simulink model "simulacao"  (R2025a)
settings: Solver=VariableStepAuto  StartTime=0.0  StopTime=50  RelTol=1e-3
undefined symbols (not defined in the file): b, g, J, l, m, Tc, theta0_rad
settings Model: Creator=luiza  LastModifiedBy=luiza

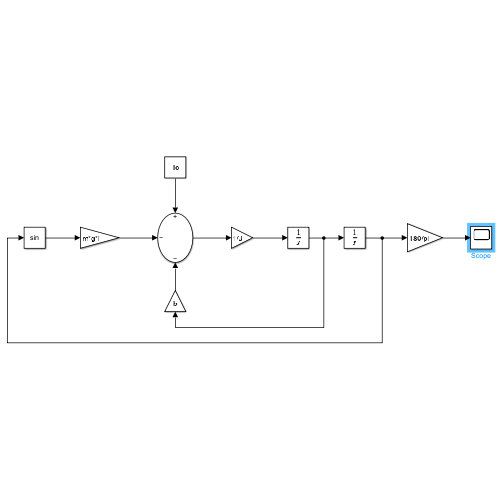
[thumbnail: Simulink's stored preview of the top-level diagram]
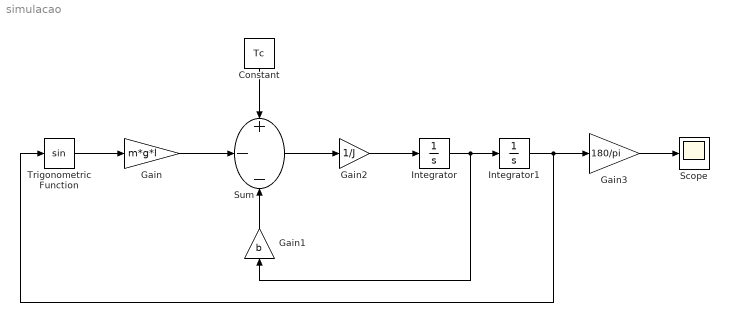
== system simulacao ==
  Constant : Constant  Value=Tc
  Gain : Gain  Gain=m*g*l
  Gain1 : Gain  Gain=b
  Gain2 : Gain  Gain=1/J
  Gain3 : Gain  Gain=180/pi
  Integrator : Integrator
  Integrator1 : Integrator  InitialCondition=theta0_rad
  Scope : Scope
      settings: ActiveDisplayYMinimum=-2.1128193962907553  ActiveDisplayYMaximum=2.8744351762193356
  Sum : Sum  Inputs=+--
  Trigonometric Function : Trigonometry
  wires:
  Constant/1 -> Sum/1
  Trigonometric Function/1 -> Gain/1
  Gain/1 -> Sum/2
  Gain1/1 -> Sum/3
  Sum/1 -> Gain2/1
  Gain2/1 -> Integrator/1
  Integrator/1 -> Gain1/1, Integrator1/1
  Integrator1/1 -> Trigonometric Function/1, Gain3/1
  Gain3/1 -> Scope/1
